simulink model "SWC_TRSP"  (R2020a)
settings: Solver=FixedStepDiscrete  StartTime=0.0  StopTime=0.15  FixedStep=0.0001  RelTol=1e-3
values from neighbouring files (symbols this model uses):
  CAL_TRSP_18VHSVoltCountTrh_s16 = 0.0    [SWC_TRSP_DataDictionary.sldd]
  CAL_TRSP_18VHSVoltDebTrh_s16 = 0.0    [SWC_TRSP_DataDictionary.sldd]
  CAL_TRSP_18VHSVoltErrRst_b = 0.0    [SWC_TRSP_DataDictionary.sldd]
  CAL_TRSP_18VHSVoltHiLim_u16 = 0.0    [SWC_TRSP_DataDictionary.sldd]
  CAL_TRSP_18VHSVoltLoLim_u16 = 0.0    [SWC_TRSP_DataDictionary.sldd]
  CAL_TRSP_1V8CPLDVoltCountTrh_s16 = 0.0    [SWC_TRSP_DataDictionary.sldd]
  CAL_TRSP_1V8CPLDVoltDebTrh_s16 = 0.0    [SWC_TRSP_DataDictionary.sldd]
  CAL_TRSP_1V8CPLDVoltErrRst_b = 0.0    [SWC_TRSP_DataDictionary.sldd]
  CAL_TRSP_1V8CPLDVoltHiLim_u16 = 0.0    [SWC_TRSP_DataDictionary.sldd]
  CAL_TRSP_1V8CPLDVoltLoLim_u16 = 0.0    [SWC_TRSP_DataDictionary.sldd]
  CAL_TRSP_3V3CPLDVoltCountTrh_s16 = 0.0    [SWC_TRSP_DataDictionary.sldd]
  CAL_TRSP_3V3CPLDVoltDebTrh_s16 = 0.0    [SWC_TRSP_DataDictionary.sldd]
  CAL_TRSP_3V3CPLDVoltErrRst_b = 0.0    [SWC_TRSP_DataDictionary.sldd]
  CAL_TRSP_3V3CPLDVoltHiLim_u16 = 0.0    [SWC_TRSP_DataDictionary.sldd]
  CAL_TRSP_3V3CPLDVoltLoLim_u16 = 0.0    [SWC_TRSP_DataDictionary.sldd]
  CAL_TRSP_AgTimecompCtl_u8 = 0.0    [SWC_TRSP_DataDictionary.sldd]
  CAL_TRSP_CurrRngCountTrh_s16 = 0.0    [SWC_TRSP_DataDictionary.sldd]
  CAL_TRSP_CurrRngDebTrh_s16 = 0.0    [SWC_TRSP_DataDictionary.sldd]
  CAL_TRSP_CurrRngErrRst_b = 0.0    [SWC_TRSP_DataDictionary.sldd]
  CAL_TRSP_CurrSumCountTrh_s16 = 0.0    [SWC_TRSP_DataDictionary.sldd]
  CAL_TRSP_CurrSumDebTrh_s16 = 0.0    [SWC_TRSP_DataDictionary.sldd]
  CAL_TRSP_CurrSumErrRst_b = 0.0    [SWC_TRSP_DataDictionary.sldd]
  CAL_TRSP_CurrSumLim_f32 = 0.0    [SWC_TRSP_DataDictionary.sldd]
  CAL_TRSP_Diff_UBR_SBCLim_f32 = 0.0    [SWC_TRSP_DataDictionary.sldd]
  CAL_TRSP_flgChangPha_b = 0.0    [SWC_TRSP_DataDictionary.sldd]
  CAL_TRSP_iPhasSensVoltCountTrh_s16 = 0.0    [SWC_TRSP_DataDictionary.sldd]
  CAL_TRSP_iPhasSensVoltDebTrh_s16 = 0.0    [SWC_TRSP_DataDictionary.sldd]
  CAL_TRSP_iPhasSensVoltErrRst_b = 0.0    [SWC_TRSP_DataDictionary.sldd]
  CAL_TRSP_iPhasSensVoltHiLim_u16 = 0.0    [SWC_TRSP_DataDictionary.sldd]
  CAL_TRSP_iPhasSensVoltLoLim_u16 = 0.0    [SWC_TRSP_DataDictionary.sldd]
  CAL_TRSP_iPhaUOffset_f32 = 0.0    [SWC_TRSP_DataDictionary.sldd]
  CAL_TRSP_iPhaVOffset_f32 = 0.0    [SWC_TRSP_DataDictionary.sldd]
  CAL_TRSP_iPhaWOffset_f32 = 0.0    [SWC_TRSP_DataDictionary.sldd]
  CAL_TRSP_iUCnvFac_f32 = 0.0    [SWC_TRSP_DataDictionary.sldd]
  CAL_TRSP_iVCnvFac_f32 = 0.0    [SWC_TRSP_DataDictionary.sldd]
  CAL_TRSP_iWCnvFac_f32 = 0.0    [SWC_TRSP_DataDictionary.sldd]
  CAL_TRSP_OfstErrRst_b = 0.0    [SWC_TRSP_DataDictionary.sldd]
  CAL_TRSP_OfstRngHiLim_f32 = 0.0    [SWC_TRSP_DataDictionary.sldd]
  CAL_TRSP_OfstRngLoLim_f32 = 0.0    [SWC_TRSP_DataDictionary.sldd]
  CAL_TRSP_ReqTrqCountTrh_s16 = 0.0    [SWC_TRSP_DataDictionary.sldd]
  CAL_TRSP_ReqTrqDebTrh_s16 = 0.0    [SWC_TRSP_DataDictionary.sldd]
  CAL_TRSP_ReqTrqErrRst_b = 0.0    [SWC_TRSP_DataDictionary.sldd]
  CAL_TRSP_ReqTrqHiLim_f32 = 0.0    [SWC_TRSP_DataDictionary.sldd]
  CAL_TRSP_ReqTrqLoLim_f32 = 0.0    [SWC_TRSP_DataDictionary.sldd]
  CAL_TRSP_RslvExciCountTrh_s16 = 0.0    [SWC_TRSP_DataDictionary.sldd]
  CAL_TRSP_RslvExciDebTrh_s16 = 0.0    [SWC_TRSP_DataDictionary.sldd]
  CAL_TRSP_RslvExciErrRst_b = 0.0    [SWC_TRSP_DataDictionary.sldd]
  CAL_TRSP_RslvMaxSele_u8 = 0.0    [SWC_TRSP_DataDictionary.sldd]
  CAL_TRSP_RslvMinSele_u8 = 0.0    [SWC_TRSP_DataDictionary.sldd]
  CAL_TRSP_RslvRngCosNHiLim_u16 = 0.0    [SWC_TRSP_DataDictionary.sldd]
  CAL_TRSP_RslvRngCosNLoLim_u16 = 0.0    [SWC_TRSP_DataDictionary.sldd]
  CAL_TRSP_RslvRngCosPHiLim_u16 = 0.0    [SWC_TRSP_DataDictionary.sldd]
  CAL_TRSP_RslvRngCosPLoLim_u16 = 0.0    [SWC_TRSP_DataDictionary.sldd]
  CAL_TRSP_RslvRngCountTrh_s16 = 0.0    [SWC_TRSP_DataDictionary.sldd]
  CAL_TRSP_RslvRngDebTrh_s16 = 0.0    [SWC_TRSP_DataDictionary.sldd]
  CAL_TRSP_RslvRngErrRst_b = 0.0    [SWC_TRSP_DataDictionary.sldd]
  CAL_TRSP_RslvRngExciHiLim_u16 = 0.0    [SWC_TRSP_DataDictionary.sldd]
  CAL_TRSP_RslvRngExciLoLim_u16 = 0.0    [SWC_TRSP_DataDictionary.sldd]
  CAL_TRSP_RslvRngSinNHiLim_u16 = 0.0    [SWC_TRSP_DataDictionary.sldd]
  CAL_TRSP_RslvRngSinNLoLim_u16 = 0.0    [SWC_TRSP_DataDictionary.sldd]
  CAL_TRSP_RslvRngSinPHiLim_u16 = 0.0    [SWC_TRSP_DataDictionary.sldd]
  CAL_TRSP_RslvRngSinPLoLim_u16 = 0.0    [SWC_TRSP_DataDictionary.sldd]
  CAL_TRSP_RslvSensVoltCountTrh_s16 = 0.0    [SWC_TRSP_DataDictionary.sldd]
  CAL_TRSP_RslvSensVoltDebTrh_s16 = 0.0    [SWC_TRSP_DataDictionary.sldd]
  CAL_TRSP_RslvSensVoltErrRst_b = 0.0    [SWC_TRSP_DataDictionary.sldd]
  CAL_TRSP_RslvSensVoltHiLim_u16 = 0.0    [SWC_TRSP_DataDictionary.sldd]
  CAL_TRSP_RslvSensVoltLoLim_u16 = 0.0    [SWC_TRSP_DataDictionary.sldd]
  CAL_TRSP_RslvSqrtCountTrh_s16 = 0.0    [SWC_TRSP_DataDictionary.sldd]
  CAL_TRSP_RslvSqrtDebTrh_s16 = 0.0    [SWC_TRSP_DataDictionary.sldd]
  CAL_TRSP_RslvSqrtErrRst_b = 0.0    [SWC_TRSP_DataDictionary.sldd]
  CAL_TRSP_RslvSqrtHiLim_u16 = 0.0    [SWC_TRSP_DataDictionary.sldd]
  CAL_TRSP_RslvSqrtLoLim_u16 = 0.0    [SWC_TRSP_DataDictionary.sldd]
  CAL_TRSP_SpeedCtlMode_u8 = 0.0    [SWC_TRSP_DataDictionary.sldd]
  CAL_TRSP_TorqueCtlMode_u8 = 0.0    [SWC_TRSP_DataDictionary.sldd]
  CAL_TRSP_UB_SBCCnvFac_f32 = 0.0    [SWC_TRSP_DataDictionary.sldd]
  CAL_TRSP_UBRVoltCountTrh_s16 = 0.0    [SWC_TRSP_DataDictionary.sldd]
  CAL_TRSP_UBRVoltDebTrh_s16 = 0.0    [SWC_TRSP_DataDictionary.sldd]
  CAL_TRSP_UBRVoltErrRst_b = 0.0    [SWC_TRSP_DataDictionary.sldd]
  CAL_TRSP_UBRWIDECnvFac_f32 = 0.0    [SWC_TRSP_DataDictionary.sldd]
  CAL_TRSP_UCurrRngHiLim_f32 = 0.0    [SWC_TRSP_DataDictionary.sldd]
  CAL_TRSP_UCurrRngLoLim_f32 = 0.0    [SWC_TRSP_DataDictionary.sldd]
  CAL_TRSP_VCurrRngHiLim_f32 = 0.0    [SWC_TRSP_DataDictionary.sldd]
  CAL_TRSP_VCurrRngLoLim_f32 = 0.0    [SWC_TRSP_DataDictionary.sldd]
  CAL_TRSP_WCurrRngHiLim_f32 = 0.0    [SWC_TRSP_DataDictionary.sldd]
  CAL_TRSP_WCurrRngLoLim_f32 = 0.0    [SWC_TRSP_DataDictionary.sldd]
  GLB_TRSP_CircAge_f32 = 0.0    [SWC_TRSP_DataDictionary.sldd]
  GLB_TRSP_MotorPole_u8 = 0.0    [SWC_TRSP_DataDictionary.sldd]
  GLB_TRSP_Sixty_f32 = 0.0    [SWC_TRSP_DataDictionary.sldd]
libraries: simulink x22
(part 10 of 13)

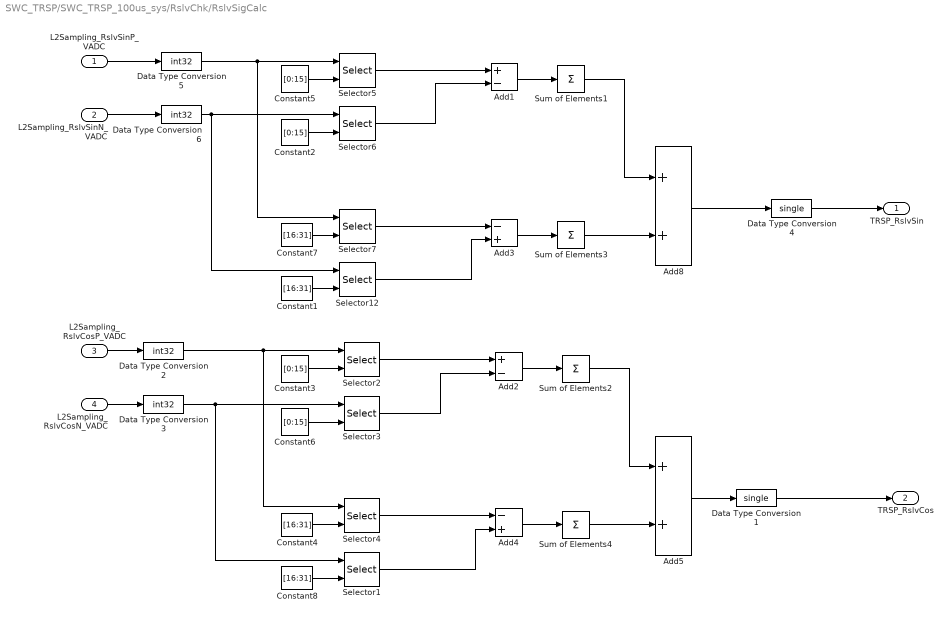
== system SWC_TRSP/SWC_TRSP_100us_sys/RslvChk/RslvSigCalc ==
  L2Sampling_RslvSinP_VADC : Inport  PortDimensions=[1 32]
  L2Sampling_RslvSinN_VADC : Inport  Port=2  PortDimensions=[1 32]
  L2Sampling_RslvCosP_VADC : Inport  Port=3  PortDimensions=[1 32]
  L2Sampling_RslvCosN_VADC : Inport  Port=4  PortDimensions=[1 32]
  Add1 : Sum  Inputs=+-
  Add2 : Sum  Inputs=+-
  Add3 : Sum  Inputs=-+
  Add4 : Sum  Inputs=-+
  Add5 : Sum
  Add8 : Sum
  Constant{1,4,7..8} (4 alike) : Constant  Value=[16:31]  OutDataTypeStr=single
  Constant{2..3,5..6} (4 alike) : Constant  Value=[0:15]  OutDataTypeStr=single
  Data Type Conversion1 : DataTypeConversion  OutDataTypeStr=single
  Data Type Conversion{2..3,5..6} (4 alike) : DataTypeConversion  OutDataTypeStr=int32
  Data Type Conversion4 : DataTypeConversion  OutDataTypeStr=single
  Selector{1..7,12} (8 alike) : Selector  IndexMode=Zero-based  InputPortWidth=32  IndexOptions=Index vector (port)  Indices=[0]  OutputSizes=1
  Sum of Elements{1..4} (4 alike) : Sum  Inputs=+
  TRSP_RslvSin : Outport
  TRSP_RslvCos : Outport  Port=2
  wires:
  L2Sampling_RslvCosP_VADC/1 -> Data Type Conversion2/1
  L2Sampling_RslvCosN_VADC/1 -> Data Type Conversion3/1
  Add5/1 -> Data Type Conversion1/1
  Data Type Conversion1/1 -> TRSP_RslvCos/1
  Data Type Conversion6/1 -> Selector12/1, Selector6/1
  Data Type Conversion5/1 -> Selector7/1, Selector5/1
  Constant2/1 -> Selector6/2
  Constant5/1 -> Selector5/2
  Selector6/1 -> Add1/2
  Selector5/1 -> Add1/1
  Add1/1 -> Sum of Elements1/1
  Sum of Elements1/1 -> Add8/1
  Add8/1 -> Data Type Conversion4/1
  Add3/1 -> Sum of Elements3/1
  Constant7/1 -> Selector7/2
  Constant1/1 -> Selector12/2
  Selector7/1 -> Add3/1
  Selector12/1 -> Add3/2
  Sum of Elements3/1 -> Add8/2
  L2Sampling_RslvSinP_VADC/1 -> Data Type Conversion5/1
  L2Sampling_RslvSinN_VADC/1 -> Data Type Conversion6/1
  Data Type Conversion4/1 -> TRSP_RslvSin/1
  Sum of Elements4/1 -> Add5/2
  Selector1/1 -> Add4/2
  Selector4/1 -> Add4/1
  Constant8/1 -> Selector1/2
  Constant4/1 -> Selector4/2
  Add4/1 -> Sum of Elements4/1
  Sum of Elements2/1 -> Add5/1
  Add2/1 -> Sum of Elements2/1
  Selector2/1 -> Add2/1
  Selector3/1 -> Add2/2
  Constant3/1 -> Selector2/2
  Constant6/1 -> Selector3/2
  Data Type Conversion2/1 -> Selector4/1, Selector2/1
  Data Type Conversion3/1 -> Selector1/1, Selector3/1

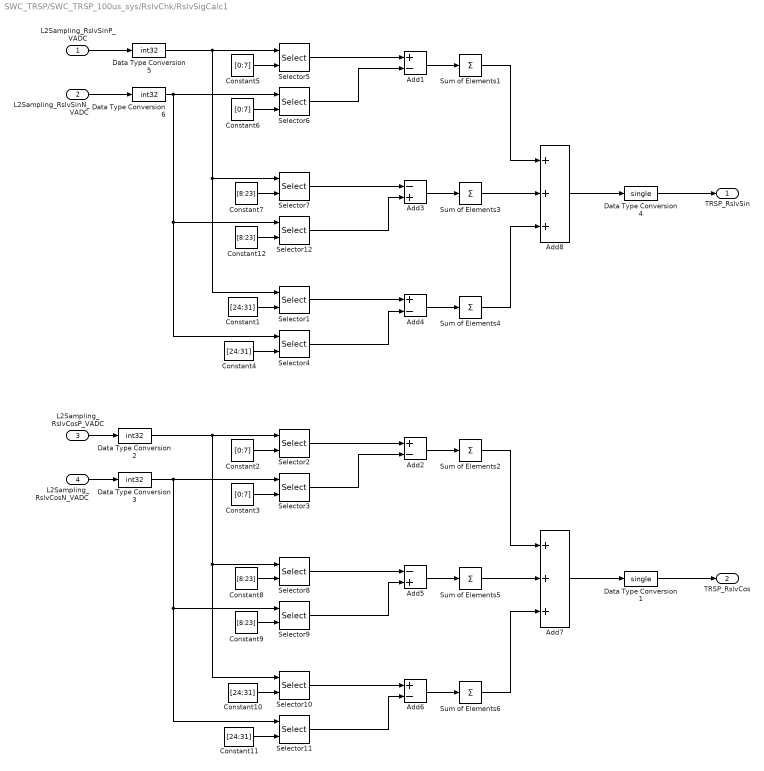
== system SWC_TRSP/SWC_TRSP_100us_sys/RslvChk/RslvSigCalc1 ==
  L2Sampling_RslvSinP_VADC : Inport  PortDimensions=[1 32]
  L2Sampling_RslvSinN_VADC : Inport  Port=2  PortDimensions=[1 32]
  L2Sampling_RslvCosP_VADC : Inport  Port=3  PortDimensions=[1 32]
  L2Sampling_RslvCosN_VADC : Inport  Port=4  PortDimensions=[1 32]
  Add{1..2,4,6} (4 alike) : Sum  Inputs=+-
  Add3 : Sum  Inputs=-+
  Add5 : Sum  Inputs=-+
  Add7 : Sum  Inputs=+++
  Add8 : Sum  Inputs=+++
  Constant{1,4,10..11} (4 alike) : Constant  Value=[24:31]  OutDataTypeStr=single
  Constant{7..9,12} (4 alike) : Constant  Value=[8:23]  OutDataTypeStr=single
  Constant{2..3,5..6} (4 alike) : Constant  Value=[0:7]  OutDataTypeStr=single
  Data Type Conversion1 : DataTypeConversion  OutDataTypeStr=single
  Data Type Conversion{2..3,5..6} (4 alike) : DataTypeConversion  OutDataTypeStr=int32
  Data Type Conversion4 : DataTypeConversion  OutDataTypeStr=single
  Selector{1..12} (12 alike) : Selector  IndexMode=Zero-based  InputPortWidth=32  IndexOptions=Index vector (port)  Indices=[0]  OutputSizes=1
  Sum of Elements{1..6} (6 alike) : Sum  Inputs=+
  TRSP_RslvSin : Outport
  TRSP_RslvCos : Outport  Port=2
  wires:
  Data Type Conversion4/1 -> TRSP_RslvSin/1
  L2Sampling_RslvSinN_VADC/1 -> Data Type Conversion6/1
  L2Sampling_RslvSinP_VADC/1 -> Data Type Conversion5/1
  Sum of Elements4/1 -> Add8/3
  Sum of Elements3/1 -> Add8/2
  Selector12/1 -> Add3/2
  Selector7/1 -> Add3/1
  Constant12/1 -> Selector12/2
  Constant7/1 -> Selector7/2
  Add3/1 -> Sum of Elements3/1
  Add4/1 -> Sum of Elements4/1
  Constant1/1 -> Selector1/2
  Constant4/1 -> Selector4/2
  Selector1/1 -> Add4/1
  Selector4/1 -> Add4/2
  Add8/1 -> Data Type Conversion4/1
  Sum of Elements1/1 -> Add8/1
  Add1/1 -> Sum of Elements1/1
  Selector5/1 -> Add1/1
  Selector6/1 -> Add1/2
  Constant5/1 -> Selector5/2
  Constant6/1 -> Selector6/2
  Data Type Conversion5/1 -> Selector5/1, Selector7/1, Selector1/1
  Data Type Conversion6/1 -> Selector6/1, Selector12/1, Selector4/1
  Data Type Conversion1/1 -> TRSP_RslvCos/1
  Data Type Conversion3/1 -> Selector11/1, Selector9/1, Selector3/1
  Data Type Conversion2/1 -> Selector10/1, Selector8/1, Selector2/1
  Constant3/1 -> Selector3/2
  Constant2/1 -> Selector2/2
  Selector3/1 -> Add2/2
  Selector2/1 -> Add2/1
  Add2/1 -> Sum of Elements2/1
  Sum of Elements2/1 -> Add7/1
  Add7/1 -> Data Type Conversion1/1
  Selector11/1 -> Add6/2
  Selector10/1 -> Add6/1
  L2Sampling_RslvCosN_VADC/1 -> Data Type Conversion3/1
  L2Sampling_RslvCosP_VADC/1 -> Data Type Conversion2/1
  Constant11/1 -> Selector11/2
  Constant10/1 -> Selector10/2
  Add6/1 -> Sum of Elements6/1
  Add5/1 -> Sum of Elements5/1
  Constant8/1 -> Selector8/2
  Constant9/1 -> Selector9/2
  Selector8/1 -> Add5/1
  Selector9/1 -> Add5/2
  Sum of Elements5/1 -> Add7/2
  Sum of Elements6/1 -> Add7/3

== system SWC_TRSP/SWC_TRSP_100us_sys/RslvChk/RslvSqrtChk ==
  TRSP_RslvSin : Inport
  TRSP_RslvCos : Inport  Port=2
  Add : Sum
  CAL_TOM_RslvSqrtLim_f1 : Constant  Value=CAL_TRSP_RslvSqrtLoLim_u16
  CAL_TOM_RslvSqrtLim_f32 : Constant  Value=CAL_TRSP_RslvSqrtHiLim_u16
  Logical Operator : Logic  Operator=OR  AllPortsSameDT=off  OutDataTypeStr=boolean
  Product : Product
  Product1 : Product
  Relational Operator : RelationalOperator  OutDataTypeStr=boolean  RndMeth=Simplest
  Relational Operator1 : RelationalOperator  Operator=<=  OutDataTypeStr=boolean  RndMeth=Simplest
  Sqrt : Sqrt  SaturateOnIntegerOverflow=on
  TRSP_RslvSqrtChkRslt : Outport
  wires:
  Product/1 -> Add/1
  TRSP_RslvSin/1 -> Product/1, Product/2
  Product1/1 -> Add/2
  CAL_TOM_RslvSqrtLim_f32/1 -> Relational Operator/2
  Sqrt/1 -> Relational Operator1/1, Relational Operator/1  "VAR_TRSP_RslvSqrt_f32"
  Add/1 -> Sqrt/1
  Relational Operator/1 -> Logical Operator/1
  TRSP_RslvCos/1 -> Product1/1, Product1/2
  CAL_TOM_RslvSqrtLim_f1/1 -> Relational Operator1/2
  Relational Operator1/1 -> Logical Operator/2
  Logical Operator/1 -> TRSP_RslvSqrtChkRslt/1

== system SWC_TRSP/SWC_TRSP_100us_sys/RslvSensVoltChk/Debouncer11 ==
  note: 1
  note: 1
  note: 0
  BooleanIN : Inport
  Rst : Inport  Port=2
  CountTrh : Inport  Port=3
  DebTrh : Inport  Port=4
  Add : Sum
  Boolean_ZERO : Constant  Value=0  OutDataTypeStr=boolean
  Compare To Zero : simulink/Logic and Bit Operations/Compare To Zero  relop===  OutDataTypeStr=boolean
  Constant : Constant  Value=0  OutDataTypeStr=int16
  Constant1 : Constant  Value=0  OutDataTypeStr=int16
  Count : Subsystem
  Delay1 : Delay  DelayLength=1
  Delay2 : Delay  DelayLength=1
  Logical Operator : Logic  Operator=OR  AllPortsSameDT=off  OutDataTypeStr=boolean
  Logical Operator1 : Logic  Operator=OR  AllPortsSameDT=off  OutDataTypeStr=boolean
  Relational Operator : RelationalOperator  OutDataTypeStr=boolean  RndMeth=Simplest
  Switch : Switch  Criteria=u2 > Threshold
  Switch1 : Switch  Criteria=u2 ~= 0
  Switch2 : Switch  Criteria=u2 > Threshold
  Unit Delay1 : UnitDelay  SampleTime=-1  HasFrameUpgradeWarning=on
  OutLock : Outport  VectorParamsAs1DForOutWhenUnconnected=off
  wires:
  Delay2/1 -> Switch2/3
  CountTrh/1 -> Count/1(CountTrh)
  Logical Operator1/1 -> Delay1/1
  Delay1/1 -> Count/Enable, Logical Operator1/1
  Switch2/1 -> Add/2
  Constant/1 -> Switch2/1
  Compare To Zero/1 -> Switch2/2
  Count/1(Count) -> Compare To Zero/1
  Logical Operator/1 -> OutLock/1, Unit Delay1/1
  Boolean_ZERO/1 -> Switch1/1
  Rst/1 -> Switch1/2
  Switch1/1 -> Logical Operator/2
  Unit Delay1/1 -> Switch1/3
  BooleanIN/1 -> Logical Operator1/2, Add/1
  Relational Operator/1 -> Switch/2, Logical Operator/1
  DebTrh/1 -> Relational Operator/2
  Switch/1 -> Delay2/1
  Add/1 -> Switch/3, Relational Operator/1
  Constant1/1 -> Switch/1

== system SWC_TRSP/SWC_TRSP_100us_sys/RslvSensVoltChk/RngChk ==
  TRSP_RngChkVal : Inport
  TRSP_HiTrh : Inport  Port=2
  TRSP_LoTrh : Inport  Port=3
  Logical Operator : Logic  Operator=OR  AllPortsSameDT=off  OutDataTypeStr=boolean
  Relational Operator : RelationalOperator  Operator=<=  OutDataTypeStr=boolean  RndMeth=Simplest
  Relational Operator1 : RelationalOperator  OutDataTypeStr=boolean  RndMeth=Simplest
  TRSP_RngChkRslt : Outport
  wires:
  Relational Operator1/1 -> Logical Operator/1
  TRSP_LoTrh/1 -> Relational Operator/2
  TRSP_RngChkVal/1 -> Relational Operator1/1, Relational Operator/1
  Logical Operator/1 -> TRSP_RngChkRslt/1
  TRSP_HiTrh/1 -> Relational Operator1/2
  Relational Operator/1 -> Logical Operator/2

== system SWC_TRSP/SWC_TRSP_100us_sys/UBRVoltChk/Debouncer11 ==
  note: 0
  note: 1
  note: 1
  BooleanIN : Inport
  Rst : Inport  Port=2
  CountTrh : Inport  Port=3
  DebTrh : Inport  Port=4
  Add : Sum
  Boolean_ZERO : Constant  Value=0  OutDataTypeStr=boolean
  Compare To Zero : simulink/Logic and Bit Operations/Compare To Zero  relop===  OutDataTypeStr=boolean
  Constant : Constant  Value=0  OutDataTypeStr=int16
  Constant1 : Constant  Value=0  OutDataTypeStr=int16
  Count : Subsystem
  Delay1 : Delay  DelayLength=1
  Delay2 : Delay  DelayLength=1
  Logical Operator : Logic  Operator=OR  AllPortsSameDT=off  OutDataTypeStr=boolean
  Logical Operator1 : Logic  Operator=OR  AllPortsSameDT=off  OutDataTypeStr=boolean
  Relational Operator : RelationalOperator  OutDataTypeStr=boolean  RndMeth=Simplest
  Switch : Switch  Criteria=u2 > Threshold
  Switch1 : Switch  Criteria=u2 ~= 0
  Switch2 : Switch  Criteria=u2 > Threshold
  Unit Delay1 : UnitDelay  SampleTime=-1  HasFrameUpgradeWarning=on
  OutLock : Outport  VectorParamsAs1DForOutWhenUnconnected=off
  wires:
  Constant1/1 -> Switch/1
  Add/1 -> Relational Operator/1, Switch/3
  Switch/1 -> Delay2/1
  DebTrh/1 -> Relational Operator/2
  Relational Operator/1 -> Logical Operator/1, Switch/2
  BooleanIN/1 -> Add/1, Logical Operator1/2
  Unit Delay1/1 -> Switch1/3
  Switch1/1 -> Logical Operator/2
  Rst/1 -> Switch1/2
  Boolean_ZERO/1 -> Switch1/1
  Logical Operator/1 -> Unit Delay1/1, OutLock/1
  Count/1(Count) -> Compare To Zero/1
  Compare To Zero/1 -> Switch2/2
  Constant/1 -> Switch2/1
  Switch2/1 -> Add/2
  Delay1/1 -> Logical Operator1/1, Count/Enable
  Logical Operator1/1 -> Delay1/1
  CountTrh/1 -> Count/1(CountTrh)
  Delay2/1 -> Switch2/3
